simulink model "PIDSch"  (R2016a)
settings: Solver=VariableStepAuto  StartTime=0.0  StopTime=10.0  RelTol=1e-3
settings Model: Creator=chenm  LastModifiedBy=chenm

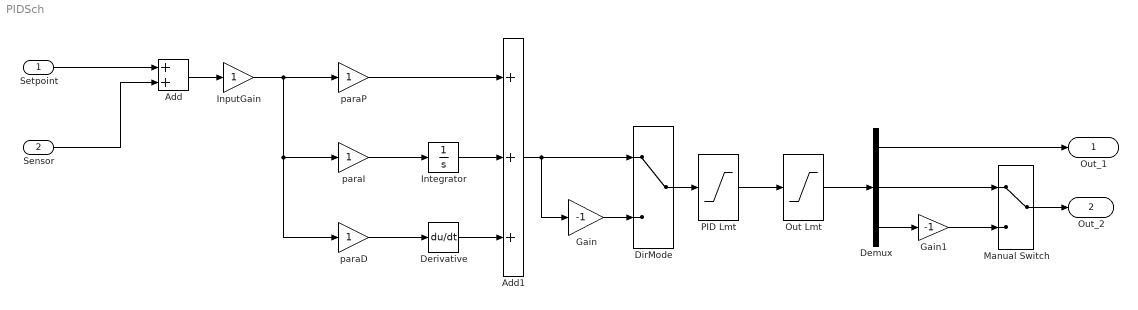
== system PIDSch ==
  Setpoint : Inport
  Sensor : Inport  Port=2
  Add : Sum
  Add1 : Sum  Inputs=+++
  Demux : Demux  Outputs=3
  Derivative : Derivative
  DirMode : ManualSwitch
  Gain : Gain  Gain=-1
  Gain1 : Gain  Gain=-1
  InputGain : Gain
  Integrator : Integrator
  Manual Switch : ManualSwitch
  Out Lmt : Saturate
  "PID Lmt　" : Saturate
  paraD : Gain
  paraI : Gain
  paraP : Gain
  "Out_1 " : Outport
  Out_2 : Outport  Port=2
  wires:
  Setpoint/1 -> Add/1
  Sensor/1 -> Add/2
  Add/1 -> InputGain/1
  InputGain/1 -> paraD/1, paraI/1, paraP/1
  paraI/1 -> Integrator/1
  paraD/1 -> Derivative/1
  paraP/1 -> Add1/1
  Integrator/1 -> Add1/2
  Derivative/1 -> Add1/3
  Add1/1 -> Gain/1, DirMode/1
  Gain/1 -> DirMode/2
  DirMode/1 -> "PID Lmt　"/1
  "PID Lmt　"/1 -> Out Lmt/1
  Out Lmt/1 -> Demux/1
  Demux/1 -> "Out_1 "/1
  Demux/2 -> Manual Switch/1
  Manual Switch/1 -> Out_2/1
  Gain1/1 -> Manual Switch/2
  Demux/3 -> Gain1/1
